simulink model "Dual_Clutch_Trans_SDO_ORIG"  (R2015b)
settings: Solver=ode1  StartTime=0.0  StopTime=15  MaxStep=0.1  RelTol=1e-3
PreLoadFcn:
  | load UrbanCycle1;
  | load UrbanCycle2;
  | load UrbanCycle3;
  | load UrbanCycle4;
  | load UrbanCycle5;
  | load UrbanCycle6;
  | load UrbanCycle7;
  | load UrbanCycle8;
  | Shift_Gear_Delay = 50;
  | Ratio_Time_Const = 0.1;
  | Drive_Cycle_Num = 7;
  | load RefRPMData;
PostLoadFcn:
  | warning off Simulink:SampleTime:TsPropEnabOutputsChangeNotAligned;
  | warning off Simulink:blocks:MatchingFromNotFound
  | warning off Simulink:blocks:MatchingGotoNotFound
  | warning off Simulink:Engine:OutputNotConnected
  | warning off Simulink:Engine:LineWithoutDst
  | warning off Simulink:Engine:UINotUpdatedDuringRapidAccelSim
  | warning off Simulink:Commands:SetParamLinkChangeWarn
  | warning off Simulink:Engine:SaveWithParameterizedLinks_Warning
undefined symbols (not defined in the file or in its folder): DCT_Param, Downshift_Speeds, sigbuilder_block, Upshift_Speeds
libraries: fl_lib x8, nesl_utility x7, sdl_lib x3, simulink x3, DCT_Vehicle_Dynamics_Lib x1
(part 2 of 2)

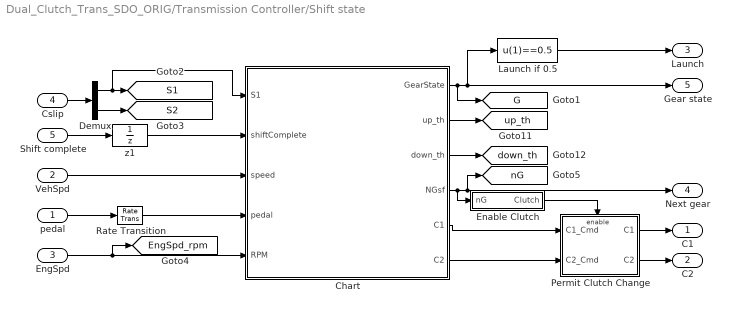
== system Dual_Clutch_Trans_SDO_ORIG/Transmission Controller/Shift state ==
  pedal : Inport
  VehSpd : Inport  Port=2
  EngSpd : Inport  Port=3
  Cslip : Inport  Port=4
  Shift complete : Inport  Port=5
  Chart : Stateflow chart  TreatAsAtomicUnit=on
  Demux : Demux  Outputs=2
  Enable Clutch : Subsystem
  Launch if 0.5 : Fcn  Expr=u(1)==0.5
  Permit Clutch Change : Subsystem  TreatAsAtomicUnit=on
  Rate Transition : RateTransition  OutPortSampleTime=0.01
  z1 : UnitDelay  SampleTime=0.01
  C1 : Outport
  C2 : Outport  Port=2
  Launch : Outport  Port=3
  Next gear : Outport  Port=4
  Gear state : Outport  Port=5
  tag scope: EngSpd_rpm=global, G=global, S1=global, S2=global, down_th=global, nG=global, up_th=global
  wires:
  VehSpd/1 -> Chart/3(speed)
  EngSpd/1 -> [EngSpd_rpm], Chart/5(RPM)
  pedal/1 -> Rate Transition/1
  Shift complete/1 -> z1/1
  z1/1 -> Chart/2(shiftComplete)
  Chart/2(up_th) -> [up_th]
  Chart/3(down_th) -> [down_th]
  Chart/4(NGsf) -> [nG], Next gear/1, Enable Clutch/1(nG)
  Chart/5(C1) -> Permit Clutch Change/1(C1_Cmd)
  Chart/6(C2) -> Permit Clutch Change/2(C2_Cmd)
  Launch if 0.5/1 -> Launch/1
  Demux/1 -> [S1], Chart/1(S1)
  Demux/2 -> [S2]
  Cslip/1 -> Demux/1
  Chart/1(GearState) -> [G], Gear state/1, Launch if 0.5/1
  Enable Clutch/1(Clutch) -> Permit Clutch Change/Enable
  Permit Clutch Change/1(C1) -> C1/1
  Permit Clutch Change/2(C2) -> C2/1
  Rate Transition/1 -> Chart/4(pedal)

== system Dual_Clutch_Trans_SDO_ORIG/Abstracted/Clutches/Odd Clutch Actuator ==
  Pdem : Inport
  Pressure controller time constant : TransferFcn  Denominator=[0.02 1]
  Simulink-PS Converter : nesl_utility/Simulink-PS Converter  PhysicalDomain=network_engine_domain  SubClassName=ps_input  LeftPortType=input  RightPortType=output  PseudoPeriodic=off  Frequencies=[]  NoiseDistribution=none  NoiseParameters=[]  Unit=Pa  AffineConversion=off  InputFiltering=off  SimscapeFilterOrder=1  InputFilterTimeConstant=.001  UdotUserProvided=0
  P : PMIOPort  Port=1  Side=Right
  wires:
  Pressure controller time constant/1 -> Simulink-PS Converter/1
  Pdem/1 -> Pressure controller time constant/1
  connections:
  P/RConn1 -- Simulink-PS Converter/RConn1

== system Dual_Clutch_Trans_SDO_ORIG/Abstracted/Clutches/Slip sensor 1 ==
  Ideal Rotational Motion Sensor : fl_lib/Mechanical/Mechanical Sensors/Ideal Rotational Motion Sensor  offset=0 rad
  PS-Simulink Converter3 : nesl_utility/PS-Simulink Converter  PhysicalDomain=network_engine_domain  SubClassName=ps_output  LeftPortType=input  RightPortType=output  PseudoPeriodic=off  Frequencies=[]  Unit=rpm  AffineConversion=off
  Zero-Order Hold : ZeroOrderHold  SampleTime=0.01
  F : PMIOPort  Port=1  Side=Right
  B : PMIOPort  Port=2  Side=Left
  S1 : Outport
  wires:
  PS-Simulink Converter3/1 -> Zero-Order Hold/1
  Zero-Order Hold/1 -> S1/1
  connections:
  Ideal Rotational Motion Sensor/RConn2 -- PS-Simulink Converter3/LConn1
  F/RConn1 -- Ideal Rotational Motion Sensor/RConn1
  B/RConn1 -- Ideal Rotational Motion Sensor/LConn1

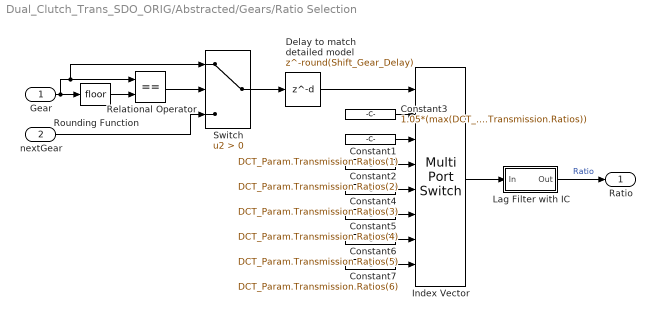
== system Dual_Clutch_Trans_SDO_ORIG/Abstracted/Gears/Ratio Selection ==
  Gear : Inport
  nextGear : Inport  Port=2
  Constant1 : Constant  Value=DCT_Param.Transmission.Ratios(1)
  Constant2 : Constant  Value=DCT_Param.Transmission.Ratios(2)
  Constant3 : Constant  Value=1.05*(max(DCT_Param.Transmission.Ratios))
  Constant4 : Constant  Value=DCT_Param.Transmission.Ratios(3)
  Constant5 : Constant  Value=DCT_Param.Transmission.Ratios(4)
  Constant6 : Constant  Value=DCT_Param.Transmission.Ratios(5)
  Constant7 : Constant  Value=DCT_Param.Transmission.Ratios(6)
  Delay to match detailed model : Delay  DelayLength=round(Shift_Gear_Delay)  InitialCondition=1  SampleTime=0.01
  Index Vector : MultiPortSwitch  DataPortOrder=Zero-based contiguous  Inputs=7  zeroidx=on
  Lag Filter with IC : Subsystem  mask(First-order lag supporting vector signals){b=Ratio_Time_Const, x_initial=DCT_Param.Transmission.Ratios(1)}
      mask prompts: b "Filter time constant"; x_initial "Initial output"
      mask help: Models a lag of the form 1/(b*s+1) where s is the Laplace operator.
  Relational Operator : RelationalOperator  Operator===  OutDataTypeStr=boolean
  Rounding Function : Rounding
  Switch : Switch  Criteria=u2 > Threshold
  Ratio : Outport
  wires:
  Delay to match detailed model/1 -> Index Vector/1
  nextGear/1 -> Switch/3
  Switch/1 -> Delay to match detailed model/1
  Relational Operator/1 -> Switch/2
  Rounding Function/1 -> Relational Operator/2
  Lag Filter with IC/1(Out) -> Ratio/1  "Ratio"
  Gear/1 -> Switch/1, Relational Operator/1, Rounding Function/1
  Constant3/1 -> Index Vector/2
  Constant1/1 -> Index Vector/3
  Constant2/1 -> Index Vector/4
  Constant4/1 -> Index Vector/5
  Constant5/1 -> Index Vector/6
  Constant6/1 -> Index Vector/7
  Constant7/1 -> Index Vector/8
  Index Vector/1 -> Lag Filter with IC/1(In)

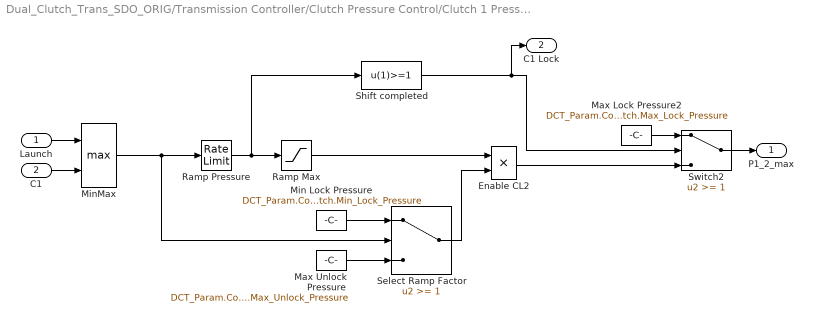
== system Dual_Clutch_Trans_SDO_ORIG/Transmission Controller/Clutch Pressure Control/Clutch 1 Pressure Gears 2 through max ==
  Launch : Inport
  C1 : Inport  Port=2
  Enable CL2 : Product  SaturateOnIntegerOverflow=on  InputSameDT=on  OutDataTypeStr=Inherit: Same as first input
  Max Lock Pressure2 : Constant  Value=DCT_Param.Control.Clutch.Max_Lock_Pressure  SampleTime=0.01
  Max Unlock Pressure : Constant  Value=DCT_Param.Control.Clutch.Max_Unlock_Pressure  SampleTime=0.01
  Min Lock Pressure : Constant  Value=DCT_Param.Control.Clutch.Min_Lock_Pressure  SampleTime=0.01
  MinMax : MinMax  Function=max  Inputs=2
  Ramp Pressure : RateLimiter  RisingSlewLimit=1/0.5  FallingSlewLimit=-1/0.5  SampleTimeMode=inherited
  Ramp Max : Saturate  UpperLimit=1/0.5  LowerLimit=0
  Select Ramp Factor : Switch  Threshold=1
  Shift completed : Fcn  Expr=u(1)>=1  SampleTime=0.01
  Switch2 : Switch  Threshold=1
  P1_2_max : Outport
  C1 Lock : Outport  Port=2
  wires:
  Launch/1 -> MinMax/1
  C1/1 -> MinMax/2
  Shift completed/1 -> Switch2/2, C1 Lock/1
  Ramp Max/1 -> Enable CL2/1
  Ramp Pressure/1 -> Ramp Max/1, Shift completed/1
  Max Unlock Pressure/1 -> Select Ramp Factor/3
  Min Lock Pressure/1 -> Select Ramp Factor/1
  Select Ramp Factor/1 -> Enable CL2/2
  Enable CL2/1 -> Switch2/3
  Max Lock Pressure2/1 -> Switch2/1
  MinMax/1 -> Select Ramp Factor/2, Ramp Pressure/1
  Switch2/1 -> P1_2_max/1

== system Dual_Clutch_Trans_SDO_ORIG/Transmission Controller/Clutch Pressure Control/Clutch 1 Pressure Launch ==
  Pedal : Inport
  Launch : Inport  Port=2
  P1_2_max : Inport  Port=3
  1/(0.18s+1) to allow for engine lag : DiscreteTransferFcn  Numerator=0.054  Denominator=[1 -0.946]  SampleTime=0.01
  Inverse clutch model : Subsystem  mask(Inverse clutch model){r_eff=0.13, N=4, A=0.001, mu=0.3}
      mask prompts: r_eff "Effective torque radius (m)"; N "Number of friction surfaces"; A "Engagement piston area (m^2)"; mu "Kinetic friction coefficient"
      mask help: Converts the demanded input torque into the required clutch pressure.
  Switch5 : Switch  Threshold=1
  Tmax : Gain  Gain=92e3/(2*pi*5500/60)  SaturateOnIntegerOverflow=on  OutDataTypeStr=Inherit: Same as input  ParamDataTypeStr=Inherit: Same as input
  P1_dem : Outport
  wires:
  Launch/1 -> Switch5/2
  Inverse clutch model/1(P) -> Switch5/1  "P_Launch"
  Pedal/1 -> Tmax/1
  1/(0.18s+1) to allow for engine lag/1 -> Inverse clutch model/1(Trq)
  Tmax/1 -> 1/(0.18s+1) to allow for engine lag/1
  Switch5/1 -> P1_dem/1
  P1_2_max/1 -> Switch5/3

== system Dual_Clutch_Trans_SDO_ORIG/Transmission Controller/Clutch Pressure Control/Clutch 2 Pressure ==
  C2 : Inport
  Enable CL : Product  SaturateOnIntegerOverflow=on  InputSameDT=on  OutDataTypeStr=Inherit: Same as first input
  Max Lock Pressure : Constant  Value=DCT_Param.Control.Clutch.Max_Lock_Pressure  SampleTime=0.01
  Max Unlock Pressure : Constant  Value=DCT_Param.Control.Clutch.Max_Unlock_Pressure  SampleTime=0.01
  Min Lock Pressure : Constant  Value=DCT_Param.Control.Clutch.Min_Lock_Pressure  SampleTime=0.01
  Ramp Pressure : RateLimiter  RisingSlewLimit=1/0.5  FallingSlewLimit=-1/0.5  SampleTimeMode=inherited
  Ramp Max1 : Saturate  UpperLimit=1/0.5  LowerLimit=0
  Rate Transition : RateTransition  OutPortSampleTime=0.01
  Select Ramp Factor : Switch  Threshold=1
  Shift completed : Fcn  Expr=u(1)>=1  SampleTime=0.01
  Switch4 : Switch  Threshold=1
  C2 Lock : Outport
  P2_dem : Outport  Port=2
  wires:
  Rate Transition/1 -> Select Ramp Factor/2, Ramp Pressure/1
  Shift completed/1 -> Switch4/2, C2 Lock/1
  Enable CL/1 -> Switch4/3
  Max Lock Pressure/1 -> Switch4/1
  Select Ramp Factor/1 -> Enable CL/2
  Min Lock Pressure/1 -> Select Ramp Factor/1
  Max Unlock Pressure/1 -> Select Ramp Factor/3
  Ramp Pressure/1 -> Shift completed/1, Ramp Max1/1
  Ramp Max1/1 -> Enable CL/1
  Switch4/1 -> P2_dem/1
  C2/1 -> Rate Transition/1

== system Dual_Clutch_Trans_SDO_ORIG/Transmission Controller/Driver/Open Loop Tests ==
  Cmd_Br : Inport
  Cmd_Pd : Inport  Port=2
  Compare To Constant : simulink/Logic and Bit Operations/Compare To Constant  relop===  const=6  OutDataTypeStr=uint8
  Demux : Demux  Outputs=2
  Open Loop Brake : Switch  Criteria=u2 > Threshold
  Open Loop Throttle : Switch  Criteria=u2 > Threshold  SampleTime=0.01
  Select Cycle : Constant  Value=Drive_Cycle_Num  SampleTime=0.01
  Step : Step  Time=[30 30]  Before=[0 1]  After=[-550 0]  SampleTime=0
  Brake : Outport
  Pedal : Outport  Port=2
  wires:
  Compare To Constant/1 -> Open Loop Brake/2, Open Loop Throttle/2
  Step/1 -> Demux/1
  Select Cycle/1 -> Compare To Constant/1
  Open Loop Brake/1 -> Brake/1  "Brake"
  Cmd_Br/1 -> Open Loop Brake/3
  Open Loop Throttle/1 -> Pedal/1  "Acc"
  Cmd_Pd/1 -> Open Loop Throttle/3
  Demux/2 -> Open Loop Throttle/1
  Demux/1 -> Open Loop Brake/1

== system Dual_Clutch_Trans_SDO_ORIG/Transmission Controller/Gear shift demands/Actuator 1 demand ==
  P : Inport
  nG : Inport  Port=2
  Disengage : Constant  Value=-1
  Engage : Constant
  Pulse sign : Switch  Threshold=0.5  InputSameDT=on
  Signed pulse : Product  SaturateOnIntegerOverflow=on  InputSameDT=on  OutDataTypeStr=Inherit: Same as first input
  Pulse : Outport
  wires:
  nG/1 -> Pulse sign/2
  P/1 -> Signed pulse/1
  Signed pulse/1 -> Pulse/1
  Pulse sign/1 -> Signed pulse/2
  Engage/1 -> Pulse sign/1
  Disengage/1 -> Pulse sign/3

== system Dual_Clutch_Trans_SDO_ORIG/Transmission Controller/Gear shift demands/Actuator 2 demand ==
  P : Inport
  nG : Inport  Port=2
  Disengage : Constant  Value=-1
  Engage : Constant
  Pulse sign : Switch  Threshold=0.5  InputSameDT=on
  Signed pulse : Product  SaturateOnIntegerOverflow=on  InputSameDT=on  OutDataTypeStr=Inherit: Same as first input
  Pulse : Outport
  wires:
  Disengage/1 -> Pulse sign/3
  Engage/1 -> Pulse sign/1
  Pulse sign/1 -> Signed pulse/2
  Signed pulse/1 -> Pulse/1
  P/1 -> Signed pulse/1
  nG/1 -> Pulse sign/2

== system Dual_Clutch_Trans_SDO_ORIG/Transmission Controller/Gear shift demands/Actuator 3 demand ==
  P : Inport
  nG : Inport  Port=2
  Disengage : Constant  Value=-1
  Engage : Constant
  Pulse sign : Switch  Threshold=0.5  InputSameDT=on
  Signed pulse : Product  SaturateOnIntegerOverflow=on  InputSameDT=on  OutDataTypeStr=Inherit: Same as first input
  Pulse : Outport
  wires:
  Disengage/1 -> Pulse sign/3
  Engage/1 -> Pulse sign/1
  Pulse sign/1 -> Signed pulse/2
  Signed pulse/1 -> Pulse/1
  P/1 -> Signed pulse/1
  nG/1 -> Pulse sign/2

== system Dual_Clutch_Trans_SDO_ORIG/Transmission Controller/Gear shift demands/Actuator 4 demand ==
  P : Inport
  nG : Inport  Port=2
  Disengage : Constant  Value=-1
  Engage : Constant
  Pulse sign : Switch  Threshold=0.5  InputSameDT=on
  Signed pulse : Product  SaturateOnIntegerOverflow=on  InputSameDT=on  OutDataTypeStr=Inherit: Same as first input
  Pulse : Outport
  wires:
  nG/1 -> Pulse sign/2
  P/1 -> Signed pulse/1
  Signed pulse/1 -> Pulse/1
  Pulse sign/1 -> Signed pulse/2
  Engage/1 -> Pulse sign/1
  Disengage/1 -> Pulse sign/3

== system Dual_Clutch_Trans_SDO_ORIG/Transmission Controller/Gear shift demands/Actuator 5 demand ==
  P : Inport
  nG : Inport  Port=2
  Disengage : Constant  Value=-1
  Engage : Constant
  Pulse sign : Switch  Threshold=0.5  InputSameDT=on
  Signed pulse : Product  SaturateOnIntegerOverflow=on  InputSameDT=on  OutDataTypeStr=Inherit: Same as first input
  Pulse : Outport
  wires:
  nG/1 -> Pulse sign/2
  P/1 -> Signed pulse/1
  Signed pulse/1 -> Pulse/1
  Pulse sign/1 -> Signed pulse/2
  Engage/1 -> Pulse sign/1
  Disengage/1 -> Pulse sign/3

== system Dual_Clutch_Trans_SDO_ORIG/Transmission Controller/Gear shift demands/Actuator 6 demand ==
  P : Inport
  nG : Inport  Port=2
  Disengage : Constant  Value=-1
  Engage : Constant
  Pulse sign : Switch  Threshold=0.5  InputSameDT=on
  Signed pulse : Product  SaturateOnIntegerOverflow=on  InputSameDT=on  OutDataTypeStr=Inherit: Same as first input
  Pulse : Outport
  wires:
  Disengage/1 -> Pulse sign/3
  Engage/1 -> Pulse sign/1
  Pulse sign/1 -> Signed pulse/2
  Signed pulse/1 -> Pulse/1
  P/1 -> Signed pulse/1
  nG/1 -> Pulse sign/2

== system Dual_Clutch_Trans_SDO_ORIG/Transmission Controller/Gear shift demands/Create pulse if next gear number changes and CL1 is not engaged ==
  ~E : Inport
  nG : Inport  Port=2
  0.5s delay : Delay  DelayLength=DCT_Param.Dog_Clutches.Pulse_Length  SampleTime=0.01
  Abs : Abs  SaturateOnIntegerOverflow=on
  Create a 1/2s pulse if not engaged and the next gear number changes : Product  SaturateOnIntegerOverflow=on  InputSameDT=on  OutDataTypeStr=Inherit: Same as first input
  Rate Transition : RateTransition  OutPortSampleTime=0.01
  Rate Transition2 : RateTransition  OutPortSampleTime=0.01
  Sum2 : Sum  Inputs=|+-  SaturateOnIntegerOverflow=on  InputSameDT=on  OutDataTypeStr=Inherit: Same as first input
  "[0,1]" : Saturate  UpperLimit=1  LowerLimit=0
  Pulse : Outport
  wires:
  Rate Transition2/1 -> 0.5s delay/1, Sum2/2
  Rate Transition/1 -> Create a 1/2s pulse if not engaged and the next gear number changes/1
  ~E/1 -> Create a 1/2s pulse if not engaged and the next gear number changes/2
  Create a 1/2s pulse if not engaged and the next gear number changes/1 -> Pulse/1
  "[0,1]"/1 -> Rate Transition/1
  Abs/1 -> "[0,1]"/1
  Sum2/1 -> Abs/1
  0.5s delay/1 -> Sum2/1
  nG/1 -> Rate Transition2/1

== system Dual_Clutch_Trans_SDO_ORIG/Transmission Controller/Gear shift demands/Create pulse if next gear number changes and CL2 is not engaged ==
  ~E : Inport
  nG : Inport  Port=2
  0.5s delay : Delay  DelayLength=DCT_Param.Dog_Clutches.Pulse_Length  SampleTime=0.01
  Abs : Abs  SaturateOnIntegerOverflow=on
  Create a 1/2s pulse if not engaged and the next gear number changes : Product  SaturateOnIntegerOverflow=on  InputSameDT=on  OutDataTypeStr=Inherit: Same as first input
  Rate Transition : RateTransition  OutPortSampleTime=0.01
  Rate Transition1 : RateTransition  OutPortSampleTime=0.01
  Sum2 : Sum  Inputs=|+-  SaturateOnIntegerOverflow=on  InputSameDT=on  OutDataTypeStr=Inherit: Same as first input
  "[0,1]" : Saturate  UpperLimit=1  LowerLimit=0
  Pulse : Outport
  wires:
  ~E/1 -> Create a 1/2s pulse if not engaged and the next gear number changes/2
  Create a 1/2s pulse if not engaged and the next gear number changes/1 -> Pulse/1
  "[0,1]"/1 -> Rate Transition/1
  Abs/1 -> "[0,1]"/1
  Sum2/1 -> Abs/1
  0.5s delay/1 -> Sum2/1
  nG/1 -> Rate Transition1/1
  Rate Transition/1 -> Create a 1/2s pulse if not engaged and the next gear number changes/1
  Rate Transition1/1 -> Sum2/2, 0.5s delay/1

== system Dual_Clutch_Trans_SDO_ORIG/Transmission Controller/Shift state/Chart/calc ==
  note: Determine if next gear will be
      | higher or lower than current gear
  gear : Inport
  pedal : Inport  Port=2
  speed : Inport  Port=3
  f : TriggerPort  TriggerType=function-call
      settings: CopyFcn=Stateflow.SLINSF.SimulinkMan.removeBlockPreDeleteFcn  PreDeleteFcn=Stateflow.SLINSF.SimulinkMan.unsafePredeleteFcn
  Add1 : Sum  Inputs=+-
  Add3 : Sum  Inputs=+-
  Add4 : Sum  Inputs=+-
  Calculate Downshift Threshold : Lookup2D  RowIndex=DCT_Param.Shift_Map.Pedal_Positions  ColumnIndex=[2,3,4,5,6]  Table=DCT_Param.Shift_Map.Downshift_Speeds  LookUpMeth=Interpolation-Use End Values
  Calculate Upshift Threshold : Lookup2D  RowIndex=Pedal_Positions  ColumnIndex=[1,2,3,4,5]  Table=Upshift_Speeds  LookUpMeth=Interpolation-Use End Values
  SpdThr : Outport
  wires:
  Add4/1 -> SpdThr/1
  Add3/1 -> Add4/2
  Add1/1 -> Add4/1
  speed/1 -> Add3/1, Add1/2
  Calculate Upshift Threshold/1 -> Add1/1
  Calculate Downshift Threshold/1 -> Add3/2
  gear/1 -> Calculate Downshift Threshold/2, Calculate Upshift Threshold/2
  pedal/1 -> Calculate Downshift Threshold/1, Calculate Upshift Threshold/1

== system Dual_Clutch_Trans_SDO_ORIG/Transmission Controller/Shift state/Chart/calc_down ==
  gear : Inport
  pedal : Inport  Port=2
  f : TriggerPort  TriggerType=function-call
      settings: CopyFcn=Stateflow.SLINSF.SimulinkMan.removeBlockPreDeleteFcn  PreDeleteFcn=Stateflow.SLINSF.SimulinkMan.unsafePredeleteFcn
  Calculate Downshift Threshold : Lookup2D  RowIndex=Pedal_Positions  ColumnIndex=[2,3,4,5,6]  Table=Downshift_Speeds  LookUpMeth=Interpolation-Use End Values
  down_th : Outport
  wires:
  pedal/1 -> Calculate Downshift Threshold/1
  gear/1 -> Calculate Downshift Threshold/2
  Calculate Downshift Threshold/1 -> down_th/1

== system Dual_Clutch_Trans_SDO_ORIG/Transmission Controller/Shift state/Chart/calc_up ==
  gear : Inport
  pedal : Inport  Port=2
  f : TriggerPort  TriggerType=function-call
      settings: CopyFcn=Stateflow.SLINSF.SimulinkMan.removeBlockPreDeleteFcn  PreDeleteFcn=Stateflow.SLINSF.SimulinkMan.unsafePredeleteFcn
  Calculate Upshift Threshold : Lookup2D  RowIndex=Pedal_Positions  ColumnIndex=[1,2,3,4,5]  Table=Upshift_Speeds  LookUpMeth=Interpolation-Use End Values
  up_th : Outport
  wires:
  gear/1 -> Calculate Upshift Threshold/2
  pedal/1 -> Calculate Upshift Threshold/1
  Calculate Upshift Threshold/1 -> up_th/1

== system Dual_Clutch_Trans_SDO_ORIG/Transmission Controller/Shift state/Enable Clutch ==
  nG : Inport
  0.5s delay : Delay  DelayLength=DCT_Param.Dog_Clutches.Pulse_Length  SampleTime=0.01
  Relational Operator : RelationalOperator  Operator===  OutDataTypeStr=boolean
  Zero-Order Hold : ZeroOrderHold  SampleTime=DCT_Param.Dog_Clutches.Pulse_Length*0.01
  Clutch : Outport
  wires:
  0.5s delay/1 -> Relational Operator/1
  Zero-Order Hold/1 -> 0.5s delay/1, Relational Operator/2
  nG/1 -> Zero-Order Hold/1
  Relational Operator/1 -> Clutch/1

== system Dual_Clutch_Trans_SDO_ORIG/Transmission Controller/Shift state/Permit Clutch Change ==
  C1_Cmd : Inport
  C2_Cmd : Inport  Port=2
  Enable : EnablePort
  C1 : Outport
  C2 : Outport  Port=2
  wires:
  C1_Cmd/1 -> C1/1
  C2_Cmd/1 -> C2/1

== system Dual_Clutch_Trans_SDO_ORIG/Abstracted/Gears/Ratio Selection/Lag Filter with IC ==
  In : Inport
  Gain : Gain  Gain=1/b
  Integrator : Integrator  InitialCondition=x_initial*b
  Sum : Sum  Inputs=|+-  SaturateOnIntegerOverflow=on  InputSameDT=on  OutDataTypeStr=Inherit: Same as first input
  Out : Outport
  wires:
  Gain/1 -> Out/1, Sum/2
  Integrator/1 -> Gain/1
  In/1 -> Sum/1
  Sum/1 -> Integrator/1

== system Dual_Clutch_Trans_SDO_ORIG/Transmission Controller/Clutch Pressure Control/Clutch 1 Pressure Launch/Inverse clutch model ==
  Trq : Inport
  Trq2P : Gain  Gain=1/(N*r_eff*mu*A)  SaturateOnIntegerOverflow=on  OutDataTypeStr=Inherit: Same as input  ParamDataTypeStr=Inherit: Same as input
  P : Outport
  wires:
  Trq2P/1 -> P/1
  Trq/1 -> Trq2P/1

== stateflow chart Dual_Clutch_Trans_SDO_ORIG/Transmission Controller/Shift state/Chart ==
  settings: sampleTime=0.01
  state GearState [parallel]
    settings: executionOrder=1
    state G1
      en: GearState=1;
      en:C1=1;C2=0;
      NGsf=2;
    state G3
      en: GearState=3;
      du:[SpdThr]=calc(3,pedal,speed);
      (history)
      state NGlow
        en: NGsf=2;
      state NGhigh
        en: NGsf=4;
      (default) -> GearState.G3.NGlow
      GearState.G3.NGlow -> GearState.G3.NGhigh : [SpdThr<0 &&...
          | GearState==3]
      GearState.G3.NGhigh -> GearState.G3.NGlow : [SpdThr>=0 &&...
          | GearState==3]
    state G2
      en: GearState=2;
      du:[SpdThr]=calc(2,pedal,speed);
      (history)
      state NGlow
        en: NGsf=1;
      state NGhigh
        en: NGsf=3;
      (default) -> GearState.G2.NGlow
      GearState.G2.NGlow -> GearState.G2.NGhigh : [SpdThr<0 &&...
          |  GearState==2]
      GearState.G2.NGhigh -> GearState.G2.NGlow : [SpdThr>=0 &&...
          |  GearState==2]
    state Launch
      en: GearState=0.5;
      en:C1=0;C2=0;
      NGsf=1;
    state G5
      en:GearState=5;
      du:[SpdThr]=calc(5,pedal,speed);
      (history)
      state NGlow
        en: NGsf=4;
      state NGhigh
        en: NGsf=6;
      (default) -> GearState.G5.NGlow
      GearState.G5.NGlow -> GearState.G5.NGhigh : [SpdThr<0 &&...
          | GearState==5]
      GearState.G5.NGhigh -> GearState.G5.NGlow : [SpdThr>=0 &&...
          | GearState==5]
    state G6
      en:GearState=6;
      NGsf=5;
    state G4
      en:GearState=4;
      du:[SpdThr]=calc(4,pedal,speed);
      (history)
      state NGlow
        en: NGsf=3;
      state NGhigh
        en: NGsf=5;
      (default) -> GearState.G4.NGlow
      GearState.G4.NGlow -> GearState.G4.NGhigh : [SpdThr<0 &&...
          | GearState==4]
      GearState.G4.NGhigh -> GearState.G4.NGlow : [SpdThr>=0 &&...
          | GearState==4]
    G1 -> G2 [order 1] : Up
    Launch -> G1 : [abs(S1)<10 && RPM>850]
        | {clutchControl=1;}
    G2 -> G3 [order 1] : Up
    G3 -> G2 [order 2] : Down
    G1 -> Launch [order 2] : [RPM<800]
        | {clutchControl=-1;}
    G2 -> G1 [order 2] : Down
    (default) -> Launch
    G3 -> G4 [order 1] : Up
    G4 -> G3 [order 2] : Down
    G4 -> G5 [order 1] : Up
    G5 -> G6 [order 1] : Up
    G6 -> G5 : Down
    G5 -> G4 [order 2] : Down
  state SelectionState [parallel]
    du:[up_th]=calc_up(GearState,pedal);
    du:[down_th]=calc_down(GearState,pedal);
    settings: executionOrder=2
    state SteadyState
      en:clutchControl=0;
    state preDownShifting
    state preUpShifting
    state UpShifting
      en: GearState=GearState+0.5;
      en:[C1,C2] = clutchstates...
      (GearState,clutchControl)
    state DownShifting
      en: GearState=GearState-0.5;
      en:[C1,C2] = clutchstates...
      (GearState,clutchControl)
    (default) -> SteadyState
    SteadyState -> (junction 62) [order 1] : [speed < down_th && ...
        | GearState >1]
        | {clutchControl=-1;}
    SteadyState -> (junction 128) [order 2] : [speed > up_th &&...
        | GearState <=5 && ...
        | floor(GearState) == GearState]
        | {clutchControl=1;}
    (junction 62) -> preDownShifting
    (junction 128) -> preUpShifting
    (junction 168) -> SteadyState
    (junction 23) -> SteadyState
    (junction 161) -> SteadyState
    preDownShifting -> (junction 168) [order 2] : [speed >= down_th]
    preUpShifting -> (junction 161) [order 2] : [speed <= up_th]
    preUpShifting -> UpShifting [order 1] : after(0.5,sec)
        | [speed>up_th]
    preDownShifting -> DownShifting [order 1] : after(0.5,sec)
        | [speed < down_th-2]
    DownShifting -> (junction 23) : [shiftComplete ==1]
        | {GearState.Down;}
    UpShifting -> (junction 23) : [shiftComplete==1]
        | {GearState.Up;}
  state up_th = calc_up(gear,pedal) [function]
  state down_th = calc_down(gear,pedal) [function]
  state SpdThr = calc(gear,pedal,speed) [function]
  data: gear function_input; pedal function_input; up_th function_output; gear function_input; pedal function_input; down_th function_output; gear function_input; pedal function_input; SpdThr function_output; speed function_input; gear function_input double; updown function_input double; cl1 function_output double; cl2 function_output double; GearState output double; S1 input; shiftComplete input; speed input; pedal input; up_th output double; down_th output double; RPM input; NGsf output double; C1 output double; C2 output double; clutchControl local double; SpdThr local double
  events: Up local EITHER_EDGE_EVENT; Down local EITHER_EDGE_EVENT
  function [cl1,cl2] = clutchstates(gear,updown):
    | function [cl1,cl2] = clutchstates(gear,updown) 
    | if (((gear==1.5)||(gear==3.5)||(gear==5.5))&&(updown==1) || ((gear==2.5)||(gear==4.5))&&(updown==-1))
    |     cl1 = 0;
    |     cl2 = 1;
    | else%if((gear==1.5)||(gear==3.5))&&(updown==-1) || ((gear==2.5)||(gear==4.5))&&(updown==1)
    | 	cl1 = 1;
    |     cl2 = 0;
    | end
